simulink library "vec_norm"  (R2025b)
settings: Solver=VariableStepAuto  StartTime=0.0  StopTime=10.0  RelTol=1e-3
settings Model: Creator=nicol  LastModifiedBy=nicol

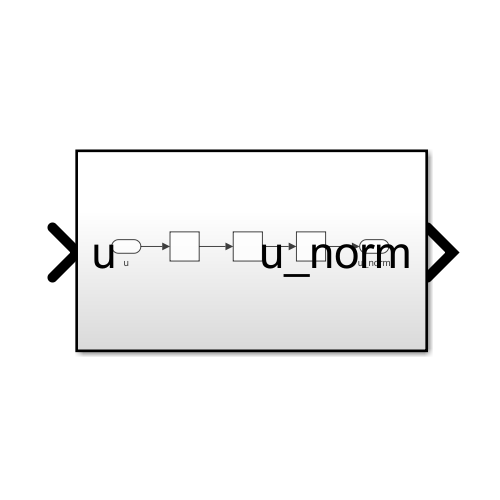
[thumbnail: Simulink's stored preview of the top-level diagram]
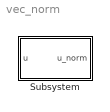
== system vec_norm ==
  Subsystem : Subsystem

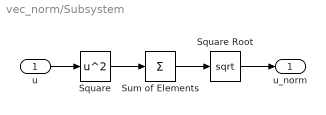
== system vec_norm/Subsystem ==
  u : Inport
  Square : Math  Operator=square
  Square Root : Sqrt
  Sum of Elements : Sum  Inputs=+
  u_norm : Outport
  wires:
  Square Root/1 -> u_norm/1
  Sum of Elements/1 -> Square Root/1
  Square/1 -> Sum of Elements/1
  u/1 -> Square/1
